simulink model "MySim4"  (R2014b)
settings: Solver=ode45  StartTime=0.0  StopTime=10.0  RelTol=1e-3
values from neighbouring files (symbols this model uses):
  K = place(A,B,PoleArray)    [script2.m]
settings Model: Creator=el12074  LastModifiedBy=gvavou5

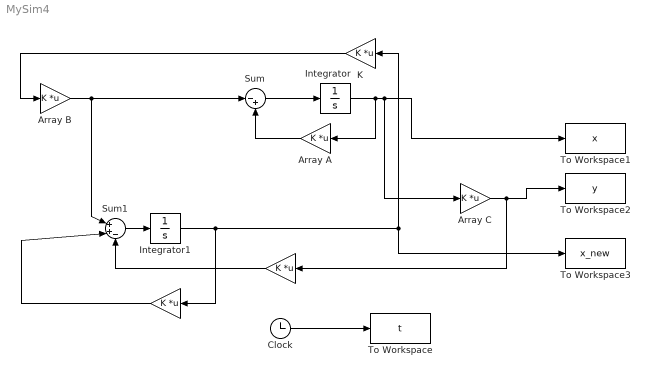
== system MySim4 ==
  " " : Gain  Gain=K  Multiplication=Matrix(K*u)
  " " : Gain  Gain=K  Multiplication=Matrix(K*u)
  Array A : Gain  Gain=K  Multiplication=Matrix(K*u)
  Array B : Gain  Gain=K  Multiplication=Matrix(K*u)
  Array C : Gain  Gain=K  Multiplication=Matrix(K*u)
  Clock : Clock
  Integrator : Integrator
  Integrator1 : Integrator
  Sum : Sum  Inputs=|-+
  Sum1 : Sum  Inputs=|++-
  To Workspace : ToWorkspace  VariableName=t  SaveFormat=Timeseries  SampleTime=-1
  To Workspace1 : ToWorkspace  VariableName=x  SaveFormat=Timeseries  SampleTime=-1
  To Workspace2 : ToWorkspace  VariableName=y  SaveFormat=Timeseries  SampleTime=-1
  To Workspace3 : ToWorkspace  VariableName=x_new  SaveFormat=Timeseries  SampleTime=-1
  Κ : Gain  Gain=K  Multiplication=Matrix(K*u)
  wires:
  Array B/1 -> Sum/1, Sum1/1
  Array A/1 -> Sum/2
  Sum/1 -> Integrator/1
  Array C/1 -> To Workspace2/1, " "/1
  Clock/1 -> To Workspace/1
  Integrator/1 -> To Workspace1/1, Array C/1, Array A/1
  " "/1 -> Sum1/3
  " "/1 -> Sum1/2
  Integrator1/1 -> To Workspace3/1, Κ/1, " "/1
  Sum1/1 -> Integrator1/1
  Κ/1 -> Array B/1
